simulink model "threebrigeconvertor6"  (Simulink 7.8)
settings: Solver=ode45  StartTime=0.0  StopTime=0.06  RelTol=1e-3
libraries: powerlib x25
settings Model: Creator=赵  LastModifiedBy=赵

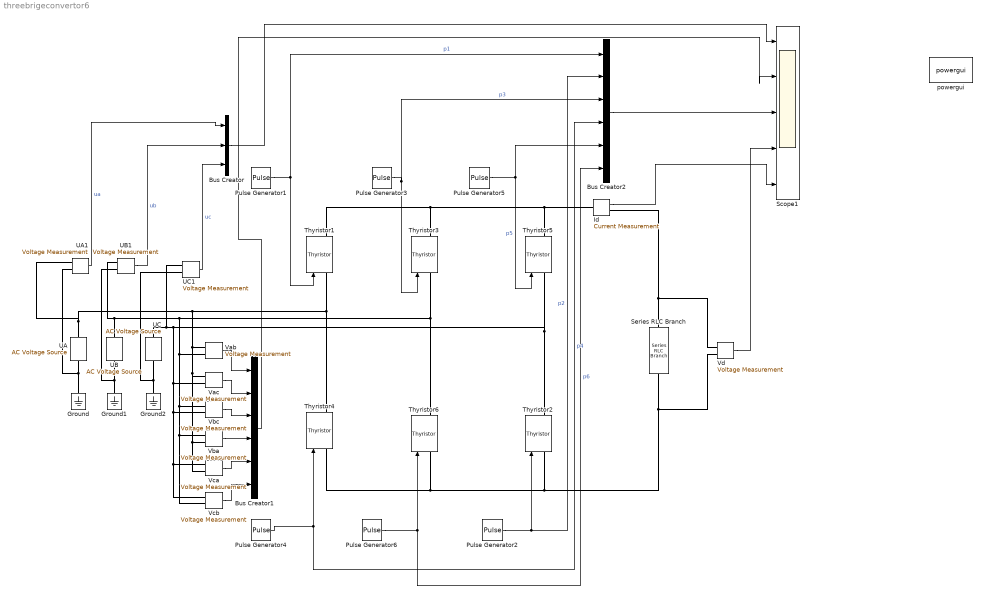
== system threebrigeconvertor6 ==
  Bus Creator : BusCreator  Inputs=3
  Bus Creator1 : BusCreator  Inputs=6
  Bus Creator2 : BusCreator  Inputs=6
  Ground : powerlib/Elements/Ground  LConnTagsString=a
  Ground1 : powerlib/Elements/Ground  LConnTagsString=a
  Ground2 : powerlib/Elements/Ground  LConnTagsString=a
  Id : powerlib/Measurements/Current Measurement  PhasorSimulation=off  OutputType=Complex  PSBequivalent=0
  Pulse Generator1 : DiscretePulseGenerator  PulseType=Time based  Amplitude=5  Period=1/50  PulseWidth=20  PhaseDelay=(60+30)/360*0.02
  Pulse Generator2 : DiscretePulseGenerator  PulseType=Time based  Amplitude=5  Period=1/50  PulseWidth=20  PhaseDelay=(60+30+60)/360*0.02
  Pulse Generator3 : DiscretePulseGenerator  PulseType=Time based  Amplitude=5  Period=1/50  PulseWidth=20  PhaseDelay=(60+30+120)/360*0.02
  Pulse Generator4 : DiscretePulseGenerator  PulseType=Time based  Amplitude=5  Period=1/50  PulseWidth=20  PhaseDelay=(60+30+180)/360*0.02
  Pulse Generator5 : DiscretePulseGenerator  PulseType=Time based  Amplitude=5  Period=1/50  PulseWidth=20  PhaseDelay=(60+30+240)/360*0.02
  Pulse Generator6 : DiscretePulseGenerator  PulseType=Time based  Amplitude=5  Period=1/50  PulseWidth=20  PhaseDelay=(60+30+300)/360*0.02
  Scope1 : Scope  NumInputPorts=5
      settings: YMin=-5~-5~-5~-5~-5  YMax=5~5~5~5~5
  Series RLC Branch : powerlib/Elements/Series RLC Branch  LConnTagsString=__new0  RConnTagsString=__new0  BranchType=RL  Resistance=2  Inductance=1e-3  SetiL0=off  InitialCurrent=0  Capacitance=1e-6  Setx0=off  InitialVoltage=0  Measurements=None
  Thyristor{1..6} (6 alike) : powerlib/Power Electronics/Thyristor  Ron=0.001  Lon=0  Vf=0.8  IC=0  Rs=500  Cs=250e-9  Measurements=on
  UA : powerlib/Electrical Sources/AC Voltage Source  Amplitude=100  Phase=0  Frequency=50  SampleTime=0  Measurements=None
  UA1 : powerlib/Measurements/Voltage Measurement  PhasorSimulation=off  OutputType=Complex  PSBequivalent=0
  UB : powerlib/Electrical Sources/AC Voltage Source  Amplitude=100  Phase=-120  Frequency=50  SampleTime=0  Measurements=None
  UB1 : powerlib/Measurements/Voltage Measurement  PhasorSimulation=off  OutputType=Complex  PSBequivalent=0
  UC : powerlib/Electrical Sources/AC Voltage Source  Amplitude=100  Phase=-240  Frequency=50  SampleTime=0  Measurements=None
  UC1 : powerlib/Measurements/Voltage Measurement  PhasorSimulation=off  OutputType=Complex  PSBequivalent=0
  Vab : powerlib/Measurements/Voltage Measurement  PhasorSimulation=off  OutputType=Complex  PSBequivalent=0
  Vac : powerlib/Measurements/Voltage Measurement  PhasorSimulation=off  OutputType=Complex  PSBequivalent=0
  Vba : powerlib/Measurements/Voltage Measurement  PhasorSimulation=off  OutputType=Complex  PSBequivalent=0
  Vbc : powerlib/Measurements/Voltage Measurement  PhasorSimulation=off  OutputType=Complex  PSBequivalent=0
  Vca : powerlib/Measurements/Voltage Measurement  PhasorSimulation=off  OutputType=Complex  PSBequivalent=0
  Vcb : powerlib/Measurements/Voltage Measurement  PhasorSimulation=off  OutputType=Complex  PSBequivalent=0
  Vd : powerlib/Measurements/Voltage Measurement  PhasorSimulation=off  OutputType=Complex  PSBequivalent=0
  powergui : powerlib/powergui  Priority=1  SimulationMode=Continuous  SolverType=Tustin  SampleTime=50e-6  frequency=60  SPID=off  DisableSnubberDevices=off  DisableRonSwitches=off  DisableVfSwitches=off  SwTol=0  Interpol=off  DisplayEquations=off  FunctionMessages=off  frequencyindice=50  Pbase=100e6  ErrMax=1e-4  Iterations=50  UnitsV=kV  UnitsW=MW  echomessages=off  HookPort=off  EnableUseOfTLC=off  x0status=blocks  RestoreLinks=warning  ResistiveCurrentMeasurement=off  Ylog=off  Xlog=on  ShowGrid=off  save=off  variable=ZData  ZoomFFT=off  StartTime=0.0  cycles=1  DisplayStyle=1  FreqAxis=off  MaxFrequency=1000  frequencyindicesteady=1  display=off  methode=off
  wires:
  Pulse Generator1/1 -> Thyristor1/1, Bus Creator2/1  "p1"
  Pulse Generator2/1 -> Thyristor2/1, Bus Creator2/2  "p2"
  Pulse Generator3/1 -> Thyristor3/1, Bus Creator2/3  "p3"
  Pulse Generator4/1 -> Thyristor4/1, Bus Creator2/4  "p4"
  Pulse Generator6/1 -> Thyristor6/1, Bus Creator2/6  "p6"
  UA1/1 -> Bus Creator/1  "ua"
  UB1/1 -> Bus Creator/2  "ub"
  UC1/1 -> Bus Creator/3  "uc"
  Vab/1 -> Bus Creator1/1
  Vac/1 -> Bus Creator1/2
  Vbc/1 -> Bus Creator1/3
  Vba/1 -> Bus Creator1/4
  Vca/1 -> Bus Creator1/5
  Vcb/1 -> Bus Creator1/6
  Pulse Generator5/1 -> Thyristor5/1, Bus Creator2/5  "p5"
  Bus Creator/1 -> Scope1/1
  Bus Creator1/1 -> Scope1/2
  Bus Creator2/1 -> Scope1/3
  Vd/1 -> Scope1/4
  Id/1 -> Scope1/5
  connections:
  Vba/LConn2 -- Thyristor4/RConn1 -- Thyristor1/LConn1 -- UA/RConn1 -- UA1/LConn1 -- Vab/LConn1 -- Vac/LConn1 -- Vca/LConn2
  Vba/LConn1 -- Vbc/LConn1 -- UB/RConn1 -- UB1/LConn1 -- Thyristor3/LConn1 -- Thyristor6/RConn1 -- Vab/LConn2 -- Vcb/LConn2
  UC/RConn1 -- UC1/LConn1 -- Thyristor2/RConn1 -- Thyristor5/LConn1 -- Vac/LConn2 -- Vbc/LConn2 -- Vca/LConn1 -- Vcb/LConn1
  Ground/LConn1 -- UA/LConn1 -- UA1/LConn2
  Ground1/LConn1 -- UB/LConn1 -- UB1/LConn2
  Ground2/LConn1 -- UC/LConn1 -- UC1/LConn2
  Thyristor5/RConn1 -- Thyristor1/RConn1 -- Thyristor3/RConn1 -- Id/LConn1
  Series RLC Branch/RConn1 -- Thyristor2/LConn1 -- Thyristor4/LConn1 -- Thyristor6/LConn1 -- Vd/LConn2
  Id/RConn1 -- Series RLC Branch/LConn1 -- Vd/LConn1
